simulink model "mdl_INS"  (R2015b)
settings: Solver=ode45  StartTime=0.0  StopTime=t_simulation  RelTol=1e-3
InitFcn:
  | launch_sim
settings Model: Creator=Adrien  LastModifiedBy=Adrien
settings DataIOCC: SaveFormat=Array
settings HardwareCC: ProdBitPerPointer=32  ProdLargestAtomicFloat=None  ProdIntDivRoundTo=Undefined  ProdEndianess=Unspecified  ProdWordSize=32  ProdHWDeviceType=32-bit Generic
settings GRTTargetCC: GeneratePreprocessorConditionals=Disable all
settings ConfigComp: CovModelRefEnable=Off

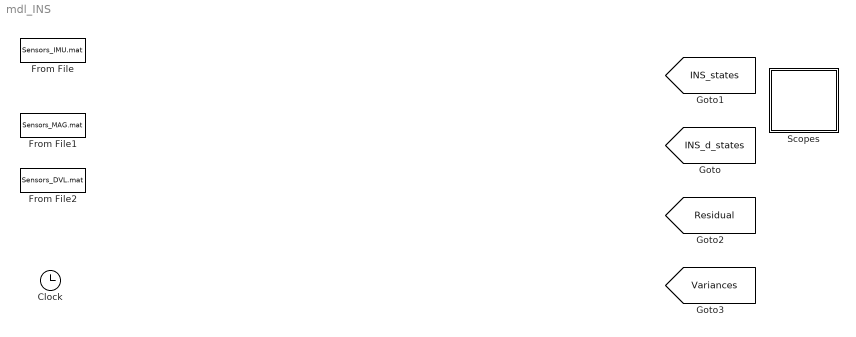
== system mdl_INS ==
  Clock : Clock
  From File : FromFile  FileName=Sensors_IMU.mat  SampleTime=0
  From File1 : FromFile  FileName=Sensors_MAG.mat  SampleTime=0
  From File2 : FromFile  FileName=Sensors_DVL.mat  SampleTime=0
  Scopes : Subsystem
  tag scope: INS_d_states=global, INS_states=global, Residual=global, Variances=global
  wires:
  ? -> [INS_d_states]
  ? -> [INS_states]
  ? -> [Residual]
  ? -> [Variances]

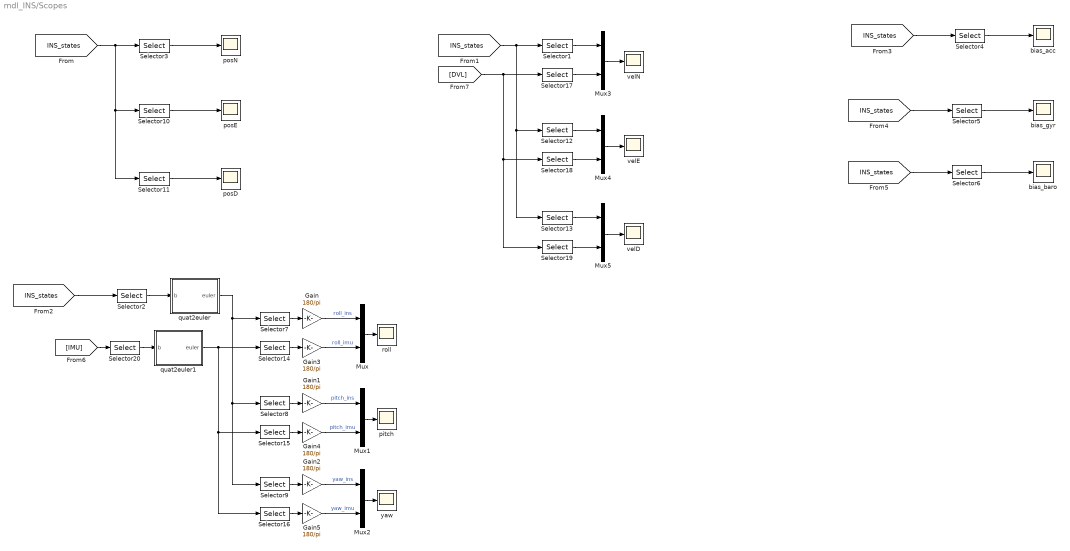
== system mdl_INS/Scopes ==
  Gain{,1..5} (6 alike) : Gain  Gain=180/pi
  Mux{,1..5} (6 alike) : Mux  Inputs=2
  Selector1 : Selector  InputPortWidth=17  IndexOptions=Index vector (dialog)  Indices=4  OutputSizes=1
  Selector10 : Selector  InputPortWidth=17  IndexOptions=Index vector (dialog)  Indices=2  OutputSizes=1
  Selector11 : Selector  InputPortWidth=17  IndexOptions=Index vector (dialog)  Indices=3  OutputSizes=1
  Selector12 : Selector  InputPortWidth=17  IndexOptions=Index vector (dialog)  Indices=5  OutputSizes=1
  Selector13 : Selector  InputPortWidth=17  IndexOptions=Index vector (dialog)  Indices=6  OutputSizes=1
  Selector14 : Selector  InputPortWidth=3  IndexOptions=Index vector (dialog)  Indices=1  OutputSizes=1
  Selector15 : Selector  InputPortWidth=3  IndexOptions=Index vector (dialog)  Indices=2  OutputSizes=1
  Selector16 : Selector  InputPortWidth=3  IndexOptions=Index vector (dialog)  Indices=3  OutputSizes=1
  Selector17 : Selector  InputPortWidth=5  IndexOptions=Index vector (dialog)  Indices=1  OutputSizes=1
  Selector18 : Selector  InputPortWidth=5  IndexOptions=Index vector (dialog)  Indices=2  OutputSizes=1
  Selector19 : Selector  InputPortWidth=5  IndexOptions=Index vector (dialog)  Indices=3  OutputSizes=1
  Selector2 : Selector  InputPortWidth=17  IndexOptions=Index vector (dialog)  Indices=[7:10]  OutputSizes=1
  Selector20 : Selector  InputPortWidth=10  IndexOptions=Index vector (dialog)  Indices=[7:10]  OutputSizes=1
  Selector3 : Selector  InputPortWidth=17  IndexOptions=Index vector (dialog)  Indices=1  OutputSizes=1
  Selector4 : Selector  InputPortWidth=17  IndexOptions=Index vector (dialog)  Indices=[11:13]  OutputSizes=1
  Selector5 : Selector  InputPortWidth=17  IndexOptions=Index vector (dialog)  Indices=[14:16]  OutputSizes=1
  Selector6 : Selector  InputPortWidth=17  IndexOptions=Index vector (dialog)  Indices=17  OutputSizes=1
  Selector7 : Selector  InputPortWidth=3  IndexOptions=Index vector (dialog)  Indices=1  OutputSizes=1
  Selector8 : Selector  InputPortWidth=3  IndexOptions=Index vector (dialog)  Indices=2  OutputSizes=1
  Selector9 : Selector  InputPortWidth=3  IndexOptions=Index vector (dialog)  Indices=3  OutputSizes=1
  bias_acc : Scope
  bias_baro : Scope
  bias_gyr : Scope
  pitch : Scope
  posD : Scope
  posE : Scope
  posN : Scope
  quat2euler : MATLAB Function  TreatAsAtomicUnit=on
  quat2euler1 : MATLAB Function  TreatAsAtomicUnit=on
  roll : Scope
  velD : Scope
  velE : Scope
  velN : Scope
  yaw : Scope
  wires:
  [INS_states] -> Selector13/1, Selector12/1, Selector1/1
  Selector2/1 -> quat2euler/1(b)
  [INS_states] -> Selector11/1, Selector10/1, Selector3/1
  Selector3/1 -> posN/1
  [INS_states] -> Selector2/1
  Selector4/1 -> bias_acc/1
  [INS_states] -> Selector4/1
  Selector5/1 -> bias_gyr/1
  [INS_states] -> Selector5/1
  Selector6/1 -> bias_baro/1
  [INS_states] -> Selector6/1
  quat2euler/1(euler) -> Selector9/1, Selector8/1, Selector7/1
  Selector8/1 -> Gain1/1
  Selector9/1 -> Gain2/1
  Selector7/1 -> Gain/1
  Selector10/1 -> posE/1
  Selector11/1 -> posD/1
  Selector14/1 -> Gain3/1
  Mux/1 -> roll/1
  Gain/1 -> Mux/1  "roll_ins"
  Mux1/1 -> pitch/1
  Mux2/1 -> yaw/1
  Gain2/1 -> Mux2/1  "yaw_ins"
  Selector15/1 -> Gain4/1
  Selector16/1 -> Gain5/1
  [IMU] -> Selector20/1
  Gain5/1 -> Mux2/2  "yaw_imu"
  Mux3/1 -> velN/1
  Selector1/1 -> Mux3/1
  [DVL] -> Selector19/1, Selector18/1, Selector17/1
  Mux4/1 -> velE/1
  Mux5/1 -> velD/1
  Selector12/1 -> Mux4/1
  Selector13/1 -> Mux5/1
  Selector17/1 -> Mux3/2
  Selector19/1 -> Mux5/2
  Selector18/1 -> Mux4/2
  Gain1/1 -> Mux1/1  "pitch_ins"
  quat2euler1/1(euler) -> Selector15/1, Selector16/1, Selector14/1
  Selector20/1 -> quat2euler1/1(b)
  Gain4/1 -> Mux1/2  "pitch_imu"
  Gain3/1 -> Mux/2  "roll_imu"

== matlab function mdl_INS/Scopes/quat2euler1 ==
  data: b input; euler output
function euler = quat2euler(b)

euler = zeros(3,1);
phi = atan2(2*(b(3)*b(4) - b(1)*b(2)),1 - 2*(b(2)^2 + b(3)^2));
theta = asin(-2*(b(2)*b(4) + b(1)*b(3)));
psi = atan2(2*(b(2)*b(3) - b(1)*b(4)),1 - 2*(b(3)^2 + b(4)^2));

euler(1) = phi;
euler(2) = theta;
euler(3) = psi;

== matlab function mdl_INS/Scopes/quat2euler ==
  data: b input; euler output
function euler = quat2euler(b)

euler = zeros(3,1);

phi = atan2(2*(b(3)*b(4) - b(1)*b(2)),1 - 2*(b(2)^2 + b(3)^2));
theta = asin(-2*(b(2)*b(4) + b(1)*b(3)));
psi = atan2(2*(b(2)*b(3) - b(1)*b(4)),1 - 2*(b(3)^2 + b(4)^2));

euler(1) = phi;
euler(2) = theta;
euler(3) = psi;
